simulink model "Taller2_SIMULINK"  (R2024a)
settings: Solver=VariableStepAuto  StartTime=0.0  StopTime=30  RelTol=1e-3
libraries: opcualib x2, sldrtlib x1
settings Model: Creator=emili  LastModifiedBy=emili

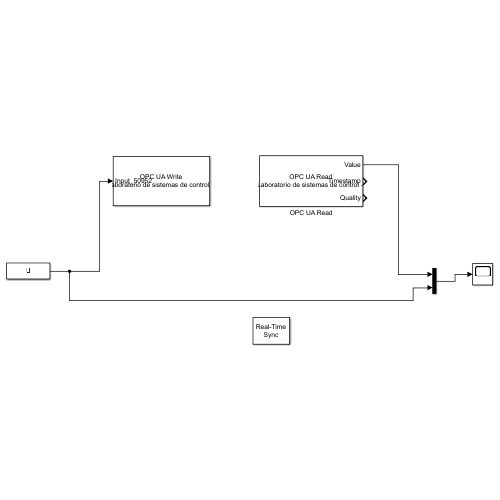
[thumbnail: Simulink's stored preview of the top-level diagram]
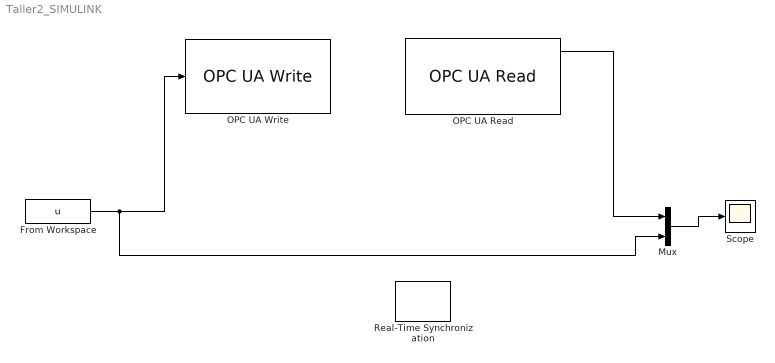
== system Taller2_SIMULINK ==
  From Workspace : FromWorkspace  VariableName=u
  Mux : Mux  Inputs=2
  OPC UA Read : opcualib/OPC UA Read  SelectedServer=UCuenca - Laboratorio de sistemas de control - open62541  ServerList=UCuenca - Laboratorio de sistemas de control - open62541  NodeList={ '1', 'Output', '0', '50953', '1' }  ShowQualityPort=on  ShowTimestampPort=on  ShowTimestampPortAs=Seconds since start  SampleTime=-1
  OPC UA Write : opcualib/OPC UA Write  SelectedServer=UCuenca - Laboratorio de sistemas de control - open62541  ServerList=UCuenca - Laboratorio de sistemas de control - open62541  SampleTime=-1  NodeList={ '1', 'Input', '0', '50952', '1' }
  Real-Time Synchronization : sldrtlib/Real-Time Synchronization  SampleTime=0.1  MaxMissedTicks=10  ShowMissedTicks=off  YieldWhenWaiting=off
  Scope : Scope
  wires:
  From Workspace/1 -> OPC UA Write/1, Mux/2
  Mux/1 -> Scope/1
  OPC UA Read/1 -> Mux/1
